simulink model "untitled"  (Simulink 9.0)
settings: Solver=VariableStepAuto  StartTime=0.0  StopTime=10.0  RelTol=1e-3
undefined symbols (not defined in the file): Dp, Dsm, g, Jp, ke, kt, Lcm, Lr, mj, ml, mr, Ra, rm
settings Model: Creator=labadmin  LastModifiedBy=The MathWorks, Inc.
settings DataIOCC: SaveFormat=Dataset
settings OptimizationCC: LifeSpan=auto
settings DebuggingCC: UnderspecifiedInitializationDetection=Simplified  MergeDetectMultiDrivingBlocksExec=error  SFUnexpectedBacktrackingDiag=error  SFNoUnconditionalDefaultTransitionDiag=error  SFExecutionAtInitializationDiag=warning
settings HardwareCC: ProdBitPerPointer=64  ProdBitPerSizeT=64  ProdBitPerPtrDiffT=64  ProdLargestAtomicFloat=Float  ProdIntDivRoundTo=Zero  ProdEndianess=LittleEndian  ProdWordSize=64  ProdHWDeviceType=Intel->x86-64 (Windows64)
settings ModelReferenceCC: PropagateSignalLabelsOutOfModel=on
settings CodeAppCC: StateflowObjectComments=off
settings GRTTargetCC: TargetLangStandard=C99 (ISO)
settings ConfigComp: CovMetricSettings=dwe  CovHtmlReporting=off  CovSaveCumulativeToWorkspaceVar=off  CovSaveSingleToWorkspaceVar=off  CovExternalEMLEnable=on

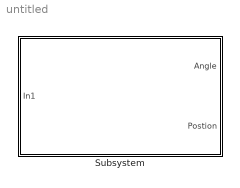
== system untitled ==
  Subsystem : Subsystem

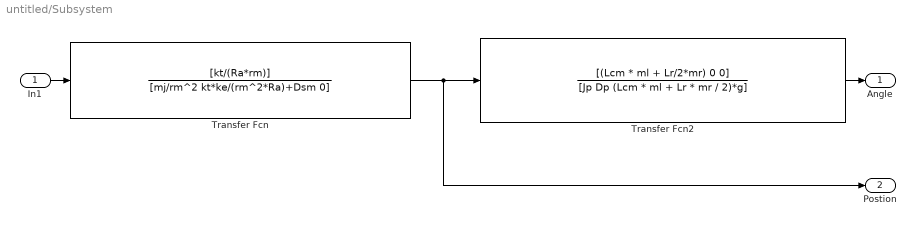
== system untitled/Subsystem ==
  In1 : Inport
  Transfer Fcn : TransferFcn  Numerator=[kt/(Ra*rm)]  Denominator=[mj/rm^2 kt*ke/(rm^2*Ra)+Dsm 0]
  Transfer Fcn2 : TransferFcn  Numerator=[(Lcm * ml + Lr/2*mr) 0 0]  Denominator=[Jp Dp (Lcm * ml + Lr * mr / 2)*g]
  Angle : Outport
  "Postion " : Outport  Port=2
  wires:
  Transfer Fcn2/1 -> Angle/1
  In1/1 -> Transfer Fcn/1
  Transfer Fcn/1 -> "Postion "/1, Transfer Fcn2/1
